simulink model "TrayectoriaStateFlow"  (R2023b)
settings: Solver=VariableStepAuto  StartTime=0.0  StopTime=10.0  RelTol=1e-3
undefined symbols (not defined in the file): d, DiscIntNeverNeededParam
settings Model: Creator=keanu  LastModifiedBy=keanu

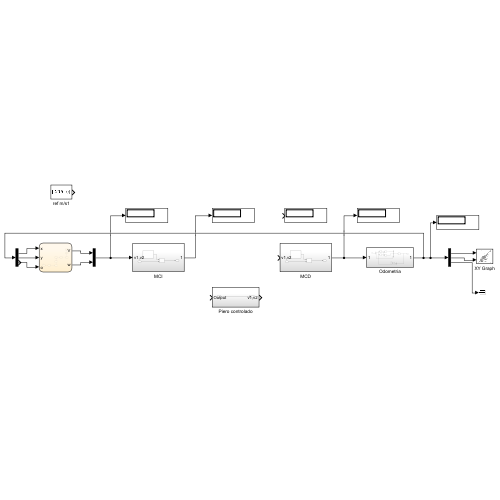
[thumbnail: Simulink's stored preview of the top-level diagram]
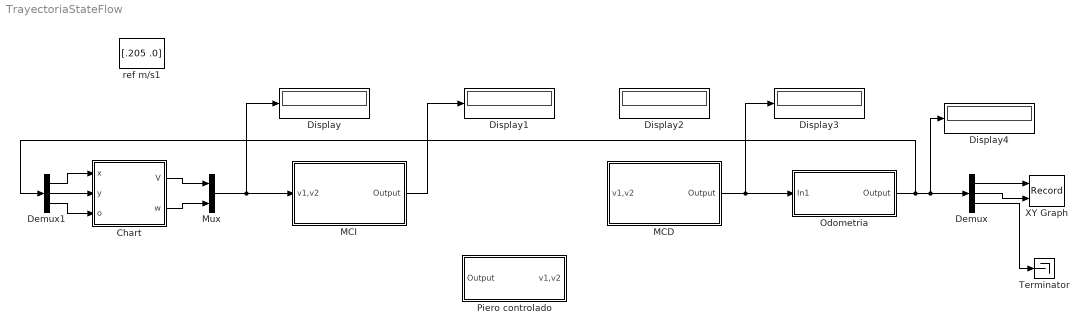
== system TrayectoriaStateFlow ==
  Chart : Stateflow chart  TreatAsAtomicUnit=on
  Demux : Demux  Outputs=3
  Demux1 : Demux  Outputs=3
  Display{,1..4} (5 alike) : Display
  MCD : Subsystem
  MCI : Subsystem
  Mux : Mux  Inputs=2
  Odometria : Subsystem
  Piero controlado : Subsystem
  Terminator : Terminator
  XY Graph : Record  FileSettingsInternal="{\"entries\":[{\"content\":{\"excelSettings\":{\"content\":{},\"type\":\"Streamout.ExcelSettings\"}},\"type\":\"Streamout.FileSettingStorage\",\"uuid\":\"\"}],\"packageUris\":[\"http:\\/\\/schema.mathworks.com\\/mf0\\/streamout_blocks\\/R2020a\"],\"version\":\"1.0\"}"  Layout=[1 1]  SignalsInternal="{\"entries\":[{\"content\":{\"signals\":[{\"content\":{\"blockPath\":[],\"dimensions\":[1],\"domain\":\"\",\"lineColor\":\"#7e2f8e\",\"port\":1,\"signalID\":1,\"signalName\":\"Demux:1\"},\"type\":\"RecordBlkView.Signal\",\"uuid\":\"\"},{\"content\":{\"blockPath\":[],\"dimensions\":[1],\"domain\":\"\",\"lineColor\":\"#77ac30\",\"port\":2,\"signalID\":2,\"signalName\":\"Demux:2\"},\"type\":\"RecordBlkView.Signal\",\"uuid\":\"\"}]},\"type\":\"RecordBlkView.InputSignals\",\"uuid\":\"\"}],\"packageUris\":[\"http:\\/\\/schema.mathworks.com\\/mf0\\/streamout_blocks\\/R2020a\"],\"version\":\"1.0\"}"  VisualizationBindings="{\"xyplotplugin\":{\"info\":[{\"series\":[],\"subplotID\":1}]}}"  CompatibilityTag=XY
  ref m/s1 : Constant  Value=[.205 .0]
  wires:
  MCD/1(Output) -> Display3/1, Odometria/1(In1)
  Mux/1 -> Display/1, MCI/1(v1,v2)
  MCI/1(Output) -> Display1/1
  Odometria/1(Output) -> Demux1/1, Display4/1, Demux/1
  Demux/1 -> XY Graph/1
  Demux/2 -> XY Graph/2
  Demux/3 -> Terminator/1
  Chart/1(V) -> Mux/1
  Chart/2(w) -> Mux/2
  Demux1/1 -> Chart/1(x)
  Demux1/2 -> Chart/2(y)
  Demux1/3 -> Chart/3(o)

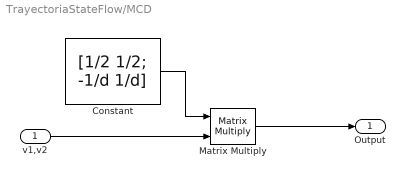
== system TrayectoriaStateFlow/MCD ==
  v1,v2 : Inport
  Constant : Constant  Value=[1/2 1/2; -1/d 1/d]
  Matrix Multiply : Product  Multiplication=Matrix(*)
  Output : Outport
  wires:
  Matrix Multiply/1 -> Output/1
  v1,v2/1 -> Matrix Multiply/2
  Constant/1 -> Matrix Multiply/1

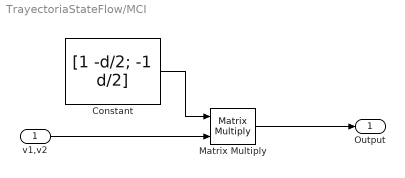
== system TrayectoriaStateFlow/MCI ==
  v1,v2 : Inport
  Constant : Constant  Value=[1 -d/2; -1 d/2]
  Matrix Multiply : Product  Multiplication=Matrix(*)
  Output : Outport
  wires:
  Constant/1 -> Matrix Multiply/1
  v1,v2/1 -> Matrix Multiply/2
  Matrix Multiply/1 -> Output/1

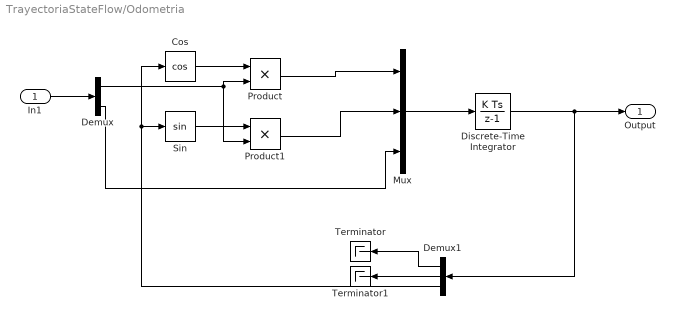
== system TrayectoriaStateFlow/Odometria ==
  In1 : Inport
  Cos : Trigonometry  Operator=cos
  Demux : Demux  Outputs=2
  Demux1 : Demux  Outputs=3
  Discrete-Time Integrator : DiscreteIntegrator  SampleTime=-1  ICPrevOutput=DiscIntNeverNeededParam  ICPrevScaledInput=DiscIntNeverNeededParam
  Mux : Mux  Inputs=3
  Product : Product
  Product1 : Product
  Sin : Trigonometry
  Terminator : Terminator
  Terminator1 : Terminator
  Output : Outport
  wires:
  Discrete-Time Integrator/1 -> Demux1/1, Output/1
  Product1/1 -> Mux/2
  In1/1 -> Demux/1
  Cos/1 -> Product/1
  Demux/2 -> Mux/3
  Demux1/3 -> Sin/1, Cos/1
  Product/1 -> Mux/1
  Demux1/2 -> Terminator1/1
  Sin/1 -> Product1/1
  Mux/1 -> Discrete-Time Integrator/1
  Demux/1 -> Product1/2, Product/2
  Demux1/1 -> Terminator/1

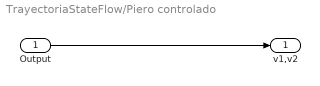
== system TrayectoriaStateFlow/Piero controlado ==
  Output : Inport
  v1,v2 : Outport
  wires:
  Output/1 -> v1,v2/1

== stateflow chart TrayectoriaStateFlow/Chart ==
  state Paro
    V=0;
    W=0;
  state Recto2
    V=0.205;
    W=0;
  state GiroDcha
    V=0.10;
    W=-pi/4;
  state Recto1
    V=0.205;
    W=0;
  state GiroIzq1
    V=0.10;
    W=pi/4;
  state Recto
    V=0.205;
    W=0;
  state Inicio
    V=0;
    W=0;
  state Marcha
    V=0.205;
    W=0;
  state GiroIzq
    V=0.10;
    W=pi/4;
  Recto2 -> Paro : [y>14]
  GiroIzq1 -> Recto2 : [o>pi/2]
  Recto1 -> GiroIzq1 : [x>3]
  GiroDcha -> Recto1 : [o>0]
  Recto -> GiroDcha : [y>12]
  GiroIzq -> Recto : [o>pi/2]
  (default) -> Inicio
  Inicio -> Marcha : [after(1,sec)]
  Marcha -> GiroIzq : [x>2.1]
  data: V output double size=1; w output double size=1; x input double size=1; y input double size=1; o input double size=1
